simulink model "Nonlinear_Model"  (R2019a)
settings: Solver=VariableStepAuto  StartTime=0.0  StopTime=10.0  RelTol=1e-3
values from neighbouring files (symbols this model uses):
  Co = 0.1285    [Setup_sim.m]
  Dp = 0.024*0    (= 0)    [Setup_sim.m]
  Dr = 0.0690    (= 0.069)    [Setup_sim.m]
  g = 0.981    [Setup_sim.m]
  init_condi = pi/180*[5, 5, 0, 0]    [Setup_sim.m]
  Jp = 0.0012    [Setup_sim.m]    (also in parameters.mat)
  Jr = 0.0083    [Setup_sim.m]    (also in parameters.mat = 0.0038)
  K_AMP = 1    [Setup_sim.m]
  Lp = 0.3111    [Setup_sim.m]    (also in parameters.mat = 0.337)
  Lr = 0.1270    (= 0.127)    [Setup_sim.m]    (also in parameters.mat)
  Mp = 0.1270    (= 0.127)    [Setup_sim.m]
  VMAX_DAC = 10    [Setup_sim.m]
undefined symbols (not defined in the file or in its folder): DiscIntNeverNeededParam, VMAX_AMP
settings Model: Creator=Ankit  LastModifiedBy=rita
settings OptimizationCC: LifeSpan=inf
settings DebuggingCC: ArithmeticOperatorsInVariantConditions=warning
settings CodeAppCC: StateflowObjectComments=on

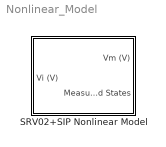
== system Nonlinear_Model ==
  SRV02+SIP Nonlinear Model : Subsystem

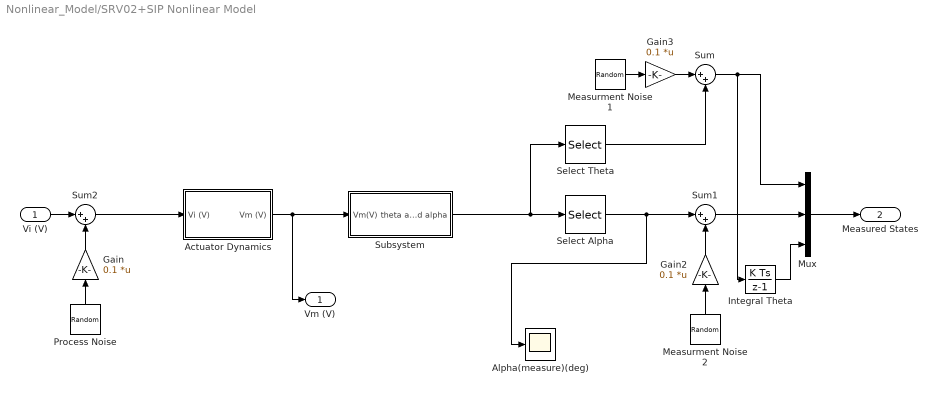
== system Nonlinear_Model/SRV02+SIP Nonlinear Model ==
  Vi (V) : Inport
  Actuator Dynamics : Subsystem
  Alpha(measure)(deg) : Scope
  Gain : Gain  Gain=0.1  Multiplication=Matrix(K*u)  SaturateOnIntegerOverflow=on  OutDataTypeStr=Inherit: Same as input  ParamDataTypeStr=Inherit: Same as input
  Gain2 : Gain  Gain=0.1  Multiplication=Matrix(K*u)  SaturateOnIntegerOverflow=on  OutDataTypeStr=Inherit: Same as input  ParamDataTypeStr=Inherit: Same as input
  Gain3 : Gain  Gain=0.1  Multiplication=Matrix(K*u)  SaturateOnIntegerOverflow=on  OutDataTypeStr=Inherit: Same as input  ParamDataTypeStr=Inherit: Same as input
  Integral Theta : DiscreteIntegrator  SampleTime=0.002  ICPrevOutput=DiscIntNeverNeededParam  ICPrevScaledInput=DiscIntNeverNeededParam
  Measurment Noise 1 : RandomNumber  Variance=0.01
  Measurment Noise 2 : RandomNumber  Variance=0.01
  Mux : Mux  Inputs=3
  Process Noise : RandomNumber  Variance=50
  Select Alpha : Selector  InputPortWidth=2  IndexOptions=Index vector (dialog)  Indices=2  OutputSizes=1
  Select Theta : Selector  InputPortWidth=2  IndexOptions=Index vector (dialog)  Indices=1  OutputSizes=1
  Subsystem : Subsystem
  Sum : Sum  Inputs=|++
  Sum1 : Sum  Inputs=|++
  Sum2 : Sum  Inputs=|++
  Vm (V) : Outport
  Measured States : Outport  Port=2
  wires:
  Actuator Dynamics/1(Vm (V)) -> Subsystem/1(Vm(V)), Vm (V)/1
  Mux/1 -> Measured States/1
  Integral Theta/1 -> Mux/3
  Select Alpha/1 -> Sum1/1, Alpha(measure)(deg)/1
  Subsystem/1(theta and alpha) -> Select Alpha/1, Select Theta/1
  Select Theta/1 -> Sum/2
  Sum/1 -> Integral Theta/1, Mux/1
  Sum1/1 -> Mux/2
  Sum2/1 -> Actuator Dynamics/1(Vi (V))
  Vi (V)/1 -> Sum2/1
  Process Noise/1 -> Gain/1
  Gain/1 -> Sum2/2
  Measurment Noise 1/1 -> Gain3/1
  Gain3/1 -> Sum/1
  Gain2/1 -> Sum1/2
  Measurment Noise 2/1 -> Gain2/1

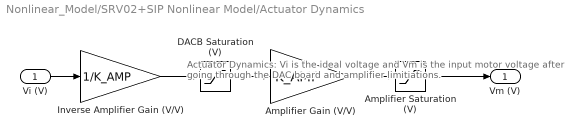
== system Nonlinear_Model/SRV02+SIP Nonlinear Model/Actuator Dynamics ==
  note: Actuator Dynamics: Vi is the ideal voltage and Vm is the
      | input motor voltage after going through the DAC board and amplifier limitiations.
  Vi (V) : Inport
  Amplifier Gain (V/V) : Gain  Gain=K_AMP
  Amplifier Saturation (V) : Saturate  UpperLimit=VMAX_AMP  LowerLimit=-VMAX_AMP
  DACB Saturation (V) : Saturate  UpperLimit=VMAX_DAC  LowerLimit=-VMAX_DAC
  Inverse Amplifier Gain (V/V) : Gain  Gain=1/K_AMP
  Vm (V) : Outport
  wires:
  Inverse Amplifier Gain (V/V)/1 -> DACB Saturation (V)/1
  DACB Saturation (V)/1 -> Amplifier Gain (V/V)/1
  Amplifier Gain (V/V)/1 -> Amplifier Saturation (V)/1
  Vi (V)/1 -> Inverse Amplifier Gain (V/V)/1
  Amplifier Saturation (V)/1 -> Vm (V)/1

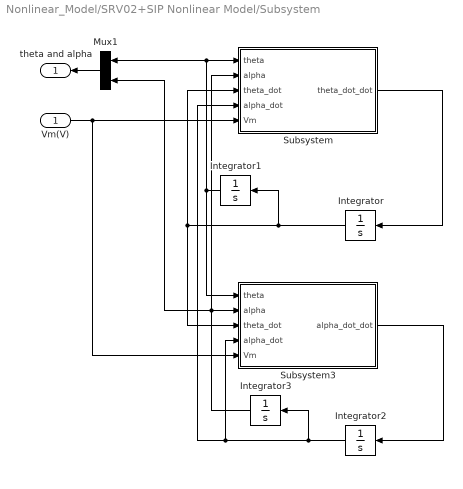
== system Nonlinear_Model/SRV02+SIP Nonlinear Model/Subsystem ==
  Vm(V) : Inport
  Integrator : Integrator  InitialCondition=init_condi(3)
  Integrator1 : Integrator  InitialCondition=init_condi(1)
  Integrator2 : Integrator  InitialCondition=init_condi(4)
  Integrator3 : Integrator  InitialCondition=init_condi(2)
  Mux1 : Mux  Inputs=2
  Subsystem : Subsystem
  Subsystem3 : Subsystem
  theta and alpha : Outport
  wires:
  Mux1/1 -> theta and alpha/1
  Integrator3/1 -> Subsystem/2(alpha), Subsystem3/2(alpha), Mux1/2
  Integrator2/1 -> Subsystem3/4(alpha_dot), Subsystem/4(alpha_dot), Integrator3/1
  Subsystem3/1(alpha_dot_dot) -> Integrator2/1
  Integrator1/1 -> Subsystem/1(theta), Mux1/1, Subsystem3/1(theta)
  Integrator/1 -> Subsystem/3(theta_dot), Subsystem3/3(theta_dot), Integrator1/1
  Subsystem/1(theta_dot_dot) -> Integrator/1
  Vm(V)/1 -> Subsystem3/5(Vm), Subsystem/5(Vm)

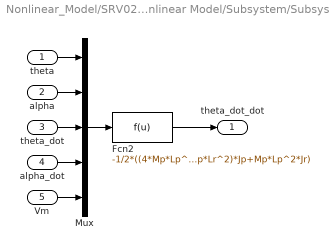
== system Nonlinear_Model/SRV02+SIP Nonlinear Model/Subsystem/Subsystem ==
  theta : Inport
  alpha : Inport  Port=2
  theta_dot : Inport  Port=3
  alpha_dot : Inport  Port=4
  Vm : Inport  Port=5
  Fcn2 : Fcn  Expr=-1/2*((4*Mp*Lp^2*u(2)*u(1)*u(4)-8*Co*u(5)+8*Dr*u(3))*Jp+(Mp^2*Lp^4*u(2)*u(3)+4*Mp*Lp*Lr*Dp)*u(4))/((4*Jr+4*Mp*Lr^2)*Jp+Mp*Lp^2*Jr)-(-1/2)*((Mp^2*Lp^3*Lr*u(3)^2+20*Mp^2*Lp^2*Lr*g)*u(2)-2*Mp*Lp^2*Dr*u(3)+2*Mp*Lp^2*Co*u(5))/((4*Jr+4*Mp*Lr^2)*Jp+Mp*Lp^2*Jr)
  Mux : Mux  Inputs=5
  theta_dot_dot : Outport
  wires:
  Fcn2/1 -> theta_dot_dot/1
  Vm/1 -> Mux/5
  alpha_dot/1 -> Mux/4
  theta_dot/1 -> Mux/3
  alpha/1 -> Mux/2
  theta/1 -> Mux/1
  Mux/1 -> Fcn2/1

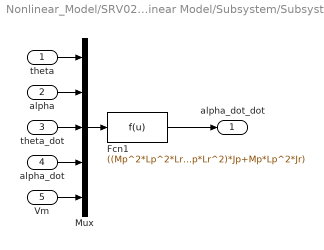
== system Nonlinear_Model/SRV02+SIP Nonlinear Model/Subsystem/Subsystem3 ==
  theta : Inport
  alpha : Inport  Port=2
  theta_dot : Inport  Port=3
  alpha_dot : Inport  Port=4
  Vm : Inport  Port=5
  Fcn1 : Fcn  Expr=((Mp^2*Lp^2*Lr^2+Mp*Lp^2*Jr)*u(3)^2+20*Jr*Mp*Lp*g+20*Mp^2*Lr^2*Lp*g)*u(2)/((4*Jr+4*Mp*Lr^2)*Jp+Mp*Lp^2*Jr)+(2*Mp*Lr*Lp*Co*u(5)-2*Mp*Lr*Lp*Dr*u(3)-(Mp^2*Lp^3*Lr*u(2)*u(3)+4*Jr*Dp+4*Mp*Lr^2*Dp)*u(4))/((4*Jr+4*Mp*Lr^2)*Jp+Mp*Lp^2*Jr)
  Mux : Mux  Inputs=5
  alpha_dot_dot : Outport
  wires:
  Fcn1/1 -> alpha_dot_dot/1
  Vm/1 -> Mux/5
  alpha_dot/1 -> Mux/4
  theta_dot/1 -> Mux/3
  alpha/1 -> Mux/2
  theta/1 -> Mux/1
  Mux/1 -> Fcn1/1
